simulink model "thyristorhalfwaveRL"  (R2018b)
settings: Solver=VariableStepAuto  StartTime=0.0  StopTime=0.06  MaxStep=1e-4  RelTol=1e-3
undefined symbols (not defined in the file): Imag, Real
libraries: powerlib x9
settings Model: Creator=sepykian  LastModifiedBy=A.hey
settings SFSimCC: SimUseLocalCustomCode=off
settings RTWCC: RTWUseLocalCustomCode=off

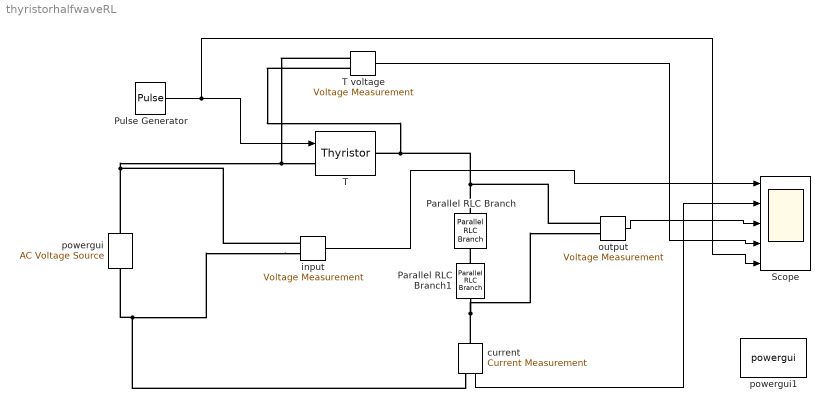
== system thyristorhalfwaveRL ==
  Parallel RLC Branch : powerlib/Elements/Parallel RLC Branch  LConnTagsString=a  RConnTagsString=__new0  BranchType=R  Resistance=134  Inductance=1e-3  SetiL0=off  InitialCurrent=0  Capacitance=1e-6  Setx0=off  InitialVoltage=0  Measurements=None
      settings: SourceProductName=Simscape Electrical
  Parallel RLC Branch1 : powerlib/Elements/Parallel RLC Branch  LConnTagsString=a  RConnTagsString=__new0  BranchType=L  Resistance=100  Inductance=1e-1  SetiL0=off  InitialCurrent=0  Capacitance=1e-6  Setx0=off  InitialVoltage=0  Measurements=None
      settings: SourceProductName=Simscape Electrical
  Pulse Generator : DiscretePulseGenerator  PulseType=Time based  Period=0.02  PulseWidth=5  PhaseDelay=0.005
  Scope : Scope  NumInputPorts=5
  T : powerlib/Power Electronics/Thyristor  Ron=0.001  Lon=0  Vf=0.8  IC=0  Rs=500  Cs=250e-9  Measurements=off
      settings: SourceProductName=Simscape Electrical
  T voltage : powerlib/Measurements/Voltage Measurement  PhasorSimulation=off  OutputType=Real-Imag  PSBequivalent=0
      settings: SourceProductName=Simscape Electrical
  current : powerlib/Measurements/Current Measurement  PhasorSimulation=off  OutputType=Real-Imag  PSBequivalent=0
      settings: SourceProductName=Simscape Electrical
  "input " : powerlib/Measurements/Voltage Measurement  PhasorSimulation=off  OutputType=Real-Imag  PSBequivalent=0
      settings: SourceProductName=Simscape Electrical
  output : powerlib/Measurements/Voltage Measurement  PhasorSimulation=off  OutputType=Real-Imag  PSBequivalent=0
      settings: SourceProductName=Simscape Electrical
  powergui : powerlib/Electrical Sources/AC Voltage Source  Amplitude=308  Phase=0  Frequency=50  SampleTime=0  Measurements=None  BusType=swing  Pref=10e3  Qref=0  Qmin=-inf  Qmax=+inf
      settings: SourceProductName=Simscape Electrical
  powergui1 : powerlib/powergui  Priority=1  SimulationMode=Continuous  SampleTime=50e-6  frequency=60  Iterations=50  frequencyindice=50  Pbase=100e6  ErrMax=1e-4  UnitsV=kV  UnitsW=MW  buscounter=0  FunctionMessages=off  echomessages=off  EnableUseOfTLC=off  CurrentSourceSwitches=off  DisableSnubberDevices=off  DisableRonSwitches=off  DisableVfSwitches=off  DisplayEquations=off  SolverType=Tustin/Backward Euler (TBE)  Interpol=off  ExternalGateDelay=off  methode=off  Ts=100  x0status=blocks  SPID=on  SwTol=0  HookPort=off  RestoreLinks=warning  ResistiveCurrentMeasurement=off  Frange=[0:2:500]  Ylog=off  Xlog=on  ShowGrid=off  save=off  variable=ZData  structure=0  ZoomFFT=off  StartTime=0.0  cycles=1  DisplayStyle=1  fundamental=60  FreqAxis=off  MaxFrequency=1000  frequencyindicesteady=1  RmsSteady=1  display=off
      settings: SourceProductName=Simscape Electrical
  wires:
  "input "/1 -> Scope/1
  current/1 -> Scope/2
  output/1 -> Scope/3
  T voltage/1 -> Scope/4
  Pulse Generator/1 -> Scope/5, T/1
  connections:
  powergui/RConn1 -- "input "/LConn1 -- T voltage/LConn1 -- T/LConn1
  Parallel RLC Branch/LConn1 -- output/LConn1 -- T voltage/LConn2 -- T/RConn1
  "input "/LConn2 -- powergui/LConn1 -- current/RConn1
  current/LConn1 -- output/LConn2 -- Parallel RLC Branch1/RConn1
  Parallel RLC Branch1/LConn1 -- Parallel RLC Branch/RConn1
